simulink model "Reverb"  (R2020a)
settings: Solver=VariableStepAuto  StartTime=0.0  StopTime=inf  RelTol=1e-3
libraries: audiosources x1, dspsnks4 x1, dspvision x1, audioeffects x1
settings Model: Creator=Zach Jones  LastModifiedBy=Zach Jones

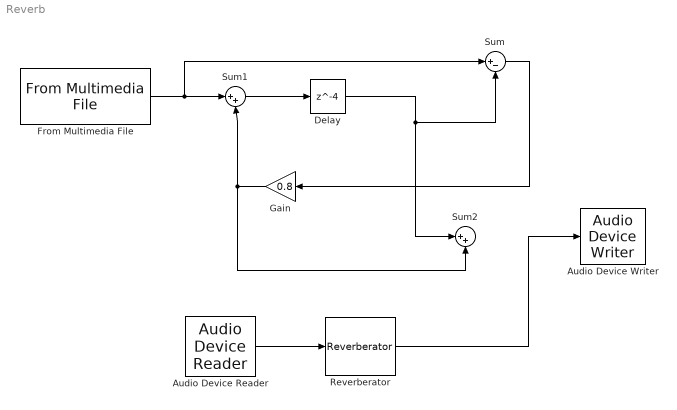
== system Reverb ==
  Audio Device Reader : audiosources/Audio Device Reader  Driver=DirectSound  Device=Microphone (iMic USB audio system)  SampleRate=44100  NumChannels=1  SamplesPerFrame=1024  BitDepth=16-bit integer  NumBuffers=10  DefaultInputChannelMapping=on  InputChannelMapping=1:2  OutputNumOverrunSamples=off  OutputDataType=double  DriverIdx=1  DeviceWarnFlag=''
      settings: SourceProductBaseCode=AU
  Audio Device Writer : dspsnks4/Audio Device Writer  Driver=DirectSound  Device=Headphones (Realtek(R) Audio)  InheritSampleRate=on  SampleRate=44100  BitDepth=16-bit integer  BufferSize=4096  NumBuffers=10  DefaultOutputChannelMapping=on  OutputChannelMapping=1:2  OutputNumUnderrunSamples=off  DriverIdx=1  DeviceWarnFlag=''
  Delay : Delay  DelayLength=4  InitialCondition=0
  From Multimedia File : dspvision/From Multimedia File  inputFilename=C:\Users\Zach Jones\Desktop\guitarTest.mp3  readRange=[1 Inf]  loop=on  numPlays=inf  outputStreams=Audio only  videoDataType=single  audioDataType=double  inheritSampleTime=on  userDefinedSampleTime=1/30  noAudioOutput=off  isIntensityVideo=off  fourcc=RGB  colorVideoFormat=Separate color signals  outputEOF=off  dataOrg=Column-major  audioFrameSize=1024  computeAudioFrameSize=off  outSamplingMode=Sample based
  Gain : Gain  Gain=0.8
  Reverberator : audioeffects/Reverberator  PreDelayPort=off  PreDelay=0.220  HighCutFrequencyPort=off  HighCutFrequency=20000  DiffusionPort=off  Diffusion=0.5  DecayFactorPort=off  DecayFactor=0.5  HighFrequencyDampingPort=off  HighFrequencyDamping=0.120  WetDryMixPort=off  WetDryMix=1.0  InheritSampleRate=on  SampleRate=44100  SimulateUsing=Interpreted execution
      settings: SourceProductBaseCode=AU
  Sum : Sum  Inputs=|+-
  Sum1 : Sum  Inputs=|++
  Sum2 : Sum  Inputs=|++
  wires:
  From Multimedia File/1 -> Sum1/1, Sum/1
  Sum1/1 -> Delay/1
  Gain/1 -> Sum2/2, Sum1/2
  Delay/1 -> Sum/2, Sum2/1
  Sum/1 -> Gain/1
  Audio Device Reader/1 -> Reverberator/1
  Reverberator/1 -> Audio Device Writer/1
